simulink model "sm_car_4post_testrig"  (R2021b)
settings: Solver=ode23t  StartTime=0.0  StopTime=20  MaxStep=0.4  RelTol=1e-3  AbsTol=1e-3  EnableMultiTasking=on
PreLoadFcn:
  | sm_car_4post_param
  | sm_car_4post_param_posts
  | load sm_car_4post_op_01
  | load sm_car_4post_op_02
  | load sm_car_4post_op_03
  | 
  | 
  | sm_car_4post_vehicle_01_data
  | sm_car_4post_vehicle_02_data
  | sm_car_4post_vehicle_03_data
  | sm_car_4post_init_data
  | Vehicle = Vehicle_01;
  | sm_car_4post_op = sm_car_4post_op_01;
values from neighbouring files (symbols this model uses):
  brake_pressure_factor = 0.1    [sm_car_4post_param.m]
  brake_rear_factor = 0.3    [sm_car_4post_param.m]
  Init = struct    [sm_car_4post_init_data.m]
  N = 100    [sm_extr_data_cam_roller_curve.m]
  s = sin(q)    [sm_extr_data_cam_roller_curve.m]
  sm_car_4post_op_01 = simscape.op.create(simlog_sm_car_4post,20)    [sm_car_4post_gen_op.m]
  Vehicle_01 = struct    [sm_car_4post_vehicle_01_data.m]
undefined symbols (not defined in the file or in its folder): Axle, Hub, ShaftF, ShaftR, smcar_param, X, xy_data_car_side, xy_data_membrane, Y, Z
libraries: fl_lib x68, sm_lib x50, nesl_utility x40, sm_car_4post_lib x34, simulink x2
(part 3 of 4)

== system sm_car_4post_testrig/Vehicle/Chassis/Body ==
  Body Geometry : Subsystem  mask(Car Body Geometry){whl_cutout_rad=whl_cutout_rad, whl_base=whl_base, thk_top=thk_top, thk_side=thk_side, car_track=car_track, extr_data_emblem_f=extr_data_emblem_f, extr_data_emblem_r=extr_data_emblem_r, clr_body_geo_top=clr_body_geo_top, opc_body_geo_top=opc_body_geo_top, clr_body_geo_left=clr_body_geo_left, opc_body_geo_left=opc_body_geo_left, clr_body_geo_right=clr_body_geo_right, opc_body_geo_right=opc_body_geo_right, clr_emblem_f=clr_emblem_f, opc_emblem_f=opc_emblem_f, clr_emblem_r=clr_emblem_r, opc_emblem_r=opc_emblem_r}
      mask prompts: whl_cutout_rad "Wheel Cutout Radius (m)"; whl_base "Wheelbase (m)"; thk_top "Top Thickness (m)"; thk_side "Side Thickness (m)"; car_track "Width (m)"; extr_data_emblem_f "Emblem Data Front [xy] (m)"; extr_data_emblem_r "Emblem Data Rear [xy] (m)"
      mask help: Creates simple car geometry. Adjusting the wheel cutout radius and wheelbase causes the profile to be adjusted. Press the Plot Profile button to see how the parameters affect the profile.
      mask init:
      | [xy_data_car_top xy_data_car_side] = sm_extr_data_car_profile(whl_cutout_rad, whl_base,thk_top);
      mask TypeOptions extr_data_emblem_f:
      | Ornament
      | Front/ExtrusionCrossSection
      mask TypeOptions extr_data_emblem_r:
      | Ornament
      | Rear/ExtrusionCrossSection
      mask TypeOptions clr_body_geo_top: Top Surface/GraphicDiffuseColor
      mask TypeOptions opc_body_geo_top: Top Surface/GraphicOpacity
      mask TypeOptions clr_body_geo_left: Left Face/GraphicDiffuseColor
      mask TypeOptions opc_body_geo_left: Left Face/GraphicOpacity
      mask TypeOptions clr_body_geo_right: Right Face/GraphicDiffuseColor
      mask TypeOptions opc_body_geo_right: Right Face/GraphicOpacity
      mask TypeOptions clr_emblem_f:
      | Ornament
      | Front/GraphicDiffuseColor
      mask TypeOptions opc_emblem_f:
      | Ornament
      | Front/GraphicOpacity
      mask TypeOptions clr_emblem_r:
      | Ornament
      | Rear/GraphicDiffuseColor
      mask TypeOptions opc_emblem_r:
      | Ornament
      | Rear/GraphicOpacity
      mask DialogControl cont_geometry Prompt: Body Geometry
      mask DialogControl push_plot_profile Prompt: Plot Profile
      mask DialogControl push_plot_profile Callback:
      | v = get_param(gcb,'MaskWSVariables');
      | getMaskValue = containers.Map({v.Name}',{v.Value}');
      | evalin('base',...
      |     sprintf('sm_extr_data_car_profile(%s,%s,%s,''%s'');',...
      |     num2str(getMaskValue('whl_cutout_rad')),...
      |     num2str(getMaskValue('whl_base')),...
      |     num2str(getMaskValue('thk_top')),'plot'));
      mask DialogControl cont_emblem Prompt: Emblem
      mask DialogControl cont_vis Prompt: Visualization
      mask DialogControl text_vis_clr Prompt: Color [RGB]
      mask DialogControl text_vis_opc Prompt: Opac. (0-1)
      mask DialogControl text_vis_top Prompt: Top
      mask DialogControl text_vis_left Prompt: Left Side
      mask DialogControl text_vis_right Prompt: Right Side
      mask DialogControl text_vis_emblem_f Prompt: Emblem Front
      mask DialogControl text_vis_emblem_r Prompt: Emblem Rear
  Body Mass and Inertia : sm_lib/Body Elements/Spherical Solid  GraphicAmbientColor=[0.15 0.15 0.15 1.0]  BasedOnType=Density  CenterOfMass=[0 0 0]  CenterOfMassUnits=m  GraphicDiffuseColor=clr_chassis_hp_cg  Density=312*0.6  DensityUnits=kg/m^3  DoExposeReferenceFrame=on  GraphicEmissiveColor=[0.0 0.0 0.0 1.0]  ExportEntireGeometry=off  SerializedExposedGeometries=<ExposedGeometries/>  SerializedFrames=<Frames/>  MarkerShape=Sphere  MarkerSize=10  GraphicType=FromGeometry  InertiaType=Custom  Mass=chassis_mass  MassUnits=kg  MomentsOfInertia=chassis_inertia  MomentsOfInertiaUnits=kg*m^2  GraphicOpacity=opc_chassis_hp_cg  ProductsOfInertia=[0 0 0]  ProductsOfInertiaUnits=kg*m^2  GraphicShininess=75  GraphicSpecularColor=[0.5 0.5 0.5 1.0]  SphereRadius=size_chassis_hp_cg  SphereRadiusUnits=m  GraphicVisPropType=SimpleVisualProperties
  Transform Body : sm_lib/Frames and Transforms/Rigid Transform  TranslationMethod=Cartesian  TranslationStandardOffset=0.4225-0.1  TranslationLengthUnit=m  TranslationStandardAxis=+Z  TranslationCartesianOffset=body_geo_hp  TranslationROffset=0  TranslationROffsetUnits=m  TranslationZOffset=0  TranslationZOffsetUnits=m  TranslationThetaOffset=0  TranslationThetaOffsetUnits=deg  RotationMethod=None  RotationAngleUnits=deg  RotationStandardAxis=+Z  RotationAngle=0.0  RotationArbitraryAxis=[0 0 1]  FollAlignAxisA=+X  BaseAlignAxisA=+Y  FollAlignAxisB=+Y  BaseAlignAxisB=+Z  RotationSequenceAxes=FollowerAxes  RotationSequence=XYX  RotationSequenceAngles=[0 0 0]  RotationSequenceAnglesUnits=deg  RotationMatrix=[1 0 0; 0 1 0; 0 0 1]
  Transform Body CG : sm_lib/Frames and Transforms/Rigid Transform  TranslationMethod=Cartesian  TranslationStandardOffset=0  TranslationLengthUnit=m  TranslationStandardAxis=+Z  TranslationCartesianOffset=hp_chassis_cg  TranslationROffset=0  TranslationROffsetUnits=m  TranslationZOffset=0  TranslationZOffsetUnits=m  TranslationThetaOffset=0  TranslationThetaOffsetUnits=deg  RotationMethod=None  RotationAngleUnits=deg  RotationStandardAxis=+Z  RotationAngle=0.0  RotationArbitraryAxis=[0 0 1]  FollAlignAxisA=+X  BaseAlignAxisA=+Y  FollAlignAxisB=+Y  BaseAlignAxisB=+Z  RotationSequenceAxes=FollowerAxes  RotationSequence=XYX  RotationSequenceAngles=[0 0 0]  RotationSequenceAnglesUnits=deg  RotationMatrix=[1 0 0; 0 1 0; 0 0 1]
  Transform Front Mount : sm_lib/Frames and Transforms/Rigid Transform  TranslationMethod=Cartesian  TranslationStandardOffset=0  TranslationLengthUnit=m  TranslationStandardAxis=+X  TranslationCartesianOffset=hp_mount_fa  TranslationROffset=0  TranslationROffsetUnits=m  TranslationZOffset=0  TranslationZOffsetUnits=m  TranslationThetaOffset=0  TranslationThetaOffsetUnits=deg  RotationMethod=None  RotationAngleUnits=deg  RotationStandardAxis=+Z  RotationAngle=0.0  RotationArbitraryAxis=[0 0 1]  FollAlignAxisA=+X  BaseAlignAxisA=+Y  FollAlignAxisB=+Y  BaseAlignAxisB=+Z  RotationSequenceAxes=FollowerAxes  RotationSequence=XYX  RotationSequenceAngles=[0 0 0]  RotationSequenceAnglesUnits=deg  RotationMatrix=[1 0 0; 0 1 0; 0 0 1]
  Transform Power Mount : sm_lib/Frames and Transforms/Rigid Transform  TranslationMethod=Cartesian  TranslationStandardOffset=0  TranslationLengthUnit=m  TranslationStandardAxis=+Z  TranslationCartesianOffset=hp_mount_power  TranslationROffset=0  TranslationROffsetUnits=m  TranslationZOffset=0  TranslationZOffsetUnits=m  TranslationThetaOffset=0  TranslationThetaOffsetUnits=deg  RotationMethod=None  RotationAngleUnits=deg  RotationStandardAxis=+Z  RotationAngle=0.0  RotationArbitraryAxis=[0 0 1]  FollAlignAxisA=+X  BaseAlignAxisA=+Y  FollAlignAxisB=+Y  BaseAlignAxisB=+Z  RotationSequenceAxes=FollowerAxes  RotationSequence=XYX  RotationSequenceAngles=[0 0 0]  RotationSequenceAnglesUnits=deg  RotationMatrix=[1 0 0; 0 1 0; 0 0 1]
  Transform Rear Mount : sm_lib/Frames and Transforms/Rigid Transform  TranslationMethod=Cartesian  TranslationStandardOffset=0  TranslationLengthUnit=m  TranslationStandardAxis=-X  TranslationCartesianOffset=hp_mount_ra  TranslationROffset=0  TranslationROffsetUnits=m  TranslationZOffset=0  TranslationZOffsetUnits=m  TranslationThetaOffset=0  TranslationThetaOffsetUnits=deg  RotationMethod=None  RotationAngleUnits=deg  RotationStandardAxis=+Z  RotationAngle=0.0  RotationArbitraryAxis=[0 0 1]  FollAlignAxisA=+X  BaseAlignAxisA=+Y  FollAlignAxisB=+Y  BaseAlignAxisB=+Z  RotationSequenceAxes=FollowerAxes  RotationSequence=XYX  RotationSequenceAngles=[0 0 0]  RotationSequenceAnglesUnits=deg  RotationMatrix=[1 0 0; 0 1 0; 0 0 1]
  Vis HP Mount Front : sm_lib/Body Elements/Spherical Solid  GraphicAmbientColor=[0.15 0.15 0.15 1.0]  BasedOnType=Density  CenterOfMass=[0 0 0]  CenterOfMassUnits=m  GraphicDiffuseColor=clr_chassis_hp_cg  Density=312*0.6  DensityUnits=kg/m^3  DoExposeReferenceFrame=on  GraphicEmissiveColor=[0.0 0.0 0.0 1.0]  ExportEntireGeometry=off  SerializedExposedGeometries=<ExposedGeometries/>  SerializedFrames=<Frames/>  MarkerShape=Sphere  MarkerSize=10  GraphicType=FromGeometry  InertiaType=PointMass  Mass=0  MassUnits=kg  MomentsOfInertia=[1 1 1]  MomentsOfInertiaUnits=kg*m^2  GraphicOpacity=opc_chassis_hp_cg  ProductsOfInertia=[0 0 0]  ProductsOfInertiaUnits=kg*m^2  GraphicShininess=75  GraphicSpecularColor=[0.5 0.5 0.5 1.0]  SphereRadius=size_chassis_hp_cg  SphereRadiusUnits=m  GraphicVisPropType=SimpleVisualProperties
  Vis HP Mount Rear : sm_lib/Body Elements/Spherical Solid  GraphicAmbientColor=[0.15 0.15 0.15 1.0]  BasedOnType=Density  CenterOfMass=[0 0 0]  CenterOfMassUnits=m  GraphicDiffuseColor=clr_chassis_hp_cg  Density=312*0.6  DensityUnits=kg/m^3  DoExposeReferenceFrame=on  GraphicEmissiveColor=[0.0 0.0 0.0 1.0]  ExportEntireGeometry=off  SerializedExposedGeometries=<ExposedGeometries/>  SerializedFrames=<Frames/>  MarkerShape=Sphere  MarkerSize=10  GraphicType=FromGeometry  InertiaType=PointMass  Mass=0  MassUnits=kg  MomentsOfInertia=[1 1 1]  MomentsOfInertiaUnits=kg*m^2  GraphicOpacity=opc_chassis_hp_cg  ProductsOfInertia=[0 0 0]  ProductsOfInertiaUnits=kg*m^2  GraphicShininess=75  GraphicSpecularColor=[0.5 0.5 0.5 1.0]  SphereRadius=size_chassis_hp_cg  SphereRadiusUnits=m  GraphicVisPropType=SimpleVisualProperties
  FA : PMIOPort  Side=Right
  Power : PMIOPort  Port=2  Side=Right
  W : PMIOPort  Port=3  Side=Left
  RA : PMIOPort  Port=4  Side=Right
  connections:
  Power/RConn1 -- Transform Power Mount/RConn1
  Transform Rear Mount/RConn1 -- Vis HP Mount Rear/RConn1 -- RA/RConn1
  FA/RConn1 -- Transform Front Mount/RConn1 -- Vis HP Mount Front/RConn1
  Body Mass and Inertia/RConn1 -- Transform Body CG/RConn1
  Transform Rear Mount/LConn1 -- Transform Power Mount/LConn1 -- Transform Front Mount/LConn1 -- W/RConn1 -- Transform Body CG/LConn1 -- Transform Body/LConn1
  Body Geometry/LConn1 -- Transform Body/RConn1

== system sm_car_4post_testrig/Vehicle/Chassis/Dampers ==
  Ctrl : Inport
  Independent : Subsystem  VariantControl=Independent
  FL : PMIOPort  Side=Left
  FR : PMIOPort  Port=2  Side=Right
  RL : PMIOPort  Port=3  Side=Left
  RR : PMIOPort  Port=4  Side=Right
  meas : Outport  VectorParamsAs1DForOutWhenUnconnected=off
  wires:
  Independent/1(meas) -> meas/1
  Ctrl/1 -> Independent/1(Ctrl)
  connections:
  Independent/RConn2 -- RR/RConn1
  Independent/RConn1 -- FR/RConn1
  Independent/LConn2 -- RL/RConn1
  Independent/LConn1 -- FL/RConn1

== system sm_car_4post_testrig/Vehicle/Chassis/Springs ==
  Ctrl : Inport
  Independent : Subsystem  VariantControl=Independent
  FL : PMIOPort  Side=Left
  FR : PMIOPort  Port=2  Side=Right
  RL : PMIOPort  Port=3  Side=Left
  RR : PMIOPort  Port=4  Side=Right
  meas : Outport  VectorParamsAs1DForOutWhenUnconnected=off
  wires:
  Independent/1(meas) -> meas/1
  Ctrl/1 -> Independent/1(Ctrl)
  connections:
  Independent/RConn2 -- RR/RConn1
  Independent/RConn1 -- FR/RConn1
  Independent/LConn1 -- FL/RConn1
  Independent/LConn2 -- RL/RConn1

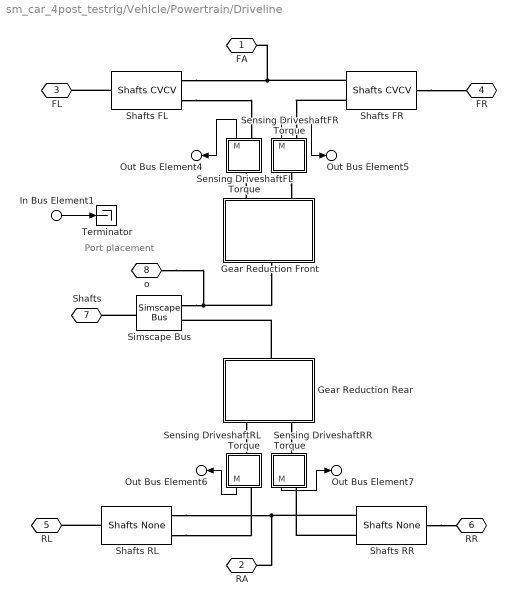
== system sm_car_4post_testrig/Vehicle/Powertrain/Driveline ==
  note: Port placement
  In Bus Element1 : Inport  PortName=CtrlBus
  Gear Reduction Front : Subsystem
  Gear Reduction Rear : Subsystem
  Sensing DriveshaftFL Torque : Subsystem
  Sensing DriveshaftFR Torque : Subsystem
  Sensing DriveshaftRL Torque : Subsystem
  Sensing DriveshaftRR Torque : Subsystem
  Shafts FL : sm_car_4post_lib/Shafts CVCV  popup_leftRight=Left  Shaft=Driveline.ShaftsFL
      settings: SourceProductBaseCode=MS
  Shafts FR : sm_car_4post_lib/Shafts CVCV  popup_leftRight=Right  Shaft=Driveline.ShaftsFR
      settings: SourceProductBaseCode=MS
  Shafts RL : sm_car_4post_lib/Shafts None  popup_leftRight=Left  Shaft=Driveline.ShaftsRL
      settings: SourceProductBaseCode=MS
  Shafts RR : sm_car_4post_lib/Shafts None  popup_leftRight=Right  Shaft=Driveline.ShaftsRR
      settings: SourceProductBaseCode=MS
  Simscape Bus : SimscapeBus  HierarchyStrings=ShaftF;ShaftR
  Terminator : Terminator
  FA : PMIOPort  Side=Left
  RA : PMIOPort  Port=2  Side=Right
  FL : PMIOPort  Port=3  Side=Left
  FR : PMIOPort  Port=4  Side=Right
  RL : PMIOPort  Port=5  Side=Left
  RR : PMIOPort  Port=6  Side=Right
  Shafts : PMIOPort  Port=7  Side=Left
  o : PMIOPort  Port=8  Side=Right
  Out Bus Element4 : Outport  VectorParamsAs1DForOutWhenUnconnected=off  PortName=DriveOut  Element=MDriveshaftFL
  Out Bus Element5 : Outport  VectorParamsAs1DForOutWhenUnconnected=off  PortName=DriveOut  Element=MDriveshaftFR
  Out Bus Element6 : Outport  VectorParamsAs1DForOutWhenUnconnected=off  PortName=DriveOut  Element=MDriveshaftRL
  Out Bus Element7 : Outport  VectorParamsAs1DForOutWhenUnconnected=off  PortName=DriveOut  Element=MDriveshaftRR
  wires:
  Sensing DriveshaftFR Torque/1(M) -> Out Bus Element5/1
  Sensing DriveshaftFL Torque/1(M) -> Out Bus Element4/1
  Sensing DriveshaftRL Torque/1(M) -> Out Bus Element6/1
  Sensing DriveshaftRR Torque/1(M) -> Out Bus Element7/1
  In Bus Element1/1 -> Terminator/1
  connections:
  Shafts FL/RConn1 -- Shafts FR/RConn1 -- FA/RConn1
  Shafts FR/LConn1 -- FR/RConn1
  Shafts RR/LConn1 -- RR/RConn1
  Shafts RL/LConn1 -- RL/RConn1
  Shafts FL/LConn1 -- FL/RConn1
  Shafts FL/RConn2 -- Sensing DriveshaftFL Torque/RConn1
  Shafts RR/RConn2 -- Sensing DriveshaftRR Torque/RConn1
  Shafts RL/RConn2 -- Sensing DriveshaftRL Torque/RConn1
  Gear Reduction Rear/LConn1 -- Simscape Bus/LConn2
  Gear Reduction Rear/RConn2 -- Sensing DriveshaftRR Torque/LConn1
  Gear Reduction Rear/RConn1 -- Sensing DriveshaftRL Torque/LConn1
  Simscape Bus/RConn1 -- Shafts/RConn1
  Shafts RL/RConn1 -- Shafts RR/RConn1 -- RA/RConn1
  Shafts FR/RConn2 -- Sensing DriveshaftFR Torque/RConn1
  o/RConn1 -- Gear Reduction Front/LConn1 -- Simscape Bus/LConn1
  Gear Reduction Front/RConn1 -- Sensing DriveshaftFL Torque/LConn1
  Sensing DriveshaftFR Torque/LConn1 -- Gear Reduction Front/RConn2

== system sm_car_4post_testrig/Vehicle/Powertrain/Power ==
  CtrlBus : Inport
  IdealTwoMotor : Subsystem  VariantControl=IdealTwoMotor  mask(Two Motor){motor_ts_f=100, motor_ts_r=100}
      mask prompts: motor_ts_f "Front Motor Cutoff Frequency (Hz)"; motor_ts_r "Rear Motor Cutoff Frequency (Hz)"
      mask help: Models two independent motors as a torque source with a simple first-order lag.
  Shafts : PMIOPort  Side=Left
  Ref : PMIOPort  Port=2  Side=Right
  PowerOut : Outport  VectorParamsAs1DForOutWhenUnconnected=off
  wires:
  IdealTwoMotor/1(PowerOut) -> PowerOut/1
  CtrlBus/1 -> IdealTwoMotor/1(CtrlBus)
  connections:
  IdealTwoMotor/RConn1 -- Ref/RConn1
  IdealTwoMotor/LConn1 -- Shafts/RConn1

== system sm_car_4post_testrig/Vehicle/Body Sensor/Roll Pitch/Calculate aPitch ==
  Roll Angle : Inport
  uvec : Inport  Port=2
  Asin : Trigonometry  Operator=asin
  Cos : Trigonometry  Operator=cos
  Divide : Product  Inputs=*/
  Divide1 : Product  Inputs=*/
  Selector : Selector  InputPortWidth=3  IndexOptions=Index vector (dialog)  Indices=[3]  OutputSizes=1
  magnitude : Fcn  Expr=sqrt(u(1)*u(1)+u(2)*u(2)+u(3)*u(3))
  Angle : Outport  VectorParamsAs1DForOutWhenUnconnected=off
  wires:
  Divide1/1 -> Asin/1
  uvec/1 -> magnitude/1, Selector/1
  magnitude/1 -> Divide1/2
  Selector/1 -> Divide/1
  Roll Angle/1 -> Cos/1
  Asin/1 -> Angle/1
  Divide/1 -> Divide1/1
  Cos/1 -> Divide/2

== system sm_car_4post_testrig/Vehicle/Body Sensor/Roll Pitch/Calculate aRoll ==
  uvec : Inport
  Demux : Demux  Outputs=3
  Mux : Mux  Inputs=2
  Trigonometric Function1 : Trigonometry  Operator=atan2
  magnitude : Fcn  Expr=sqrt(u(1)*u(1)+u(2)*u(2))
  Angle : Outport  VectorParamsAs1DForOutWhenUnconnected=off
  wires:
  Demux/2 -> Mux/2
  magnitude/1 -> Trigonometric Function1/2
  Mux/1 -> magnitude/1
  Demux/3 -> Trigonometric Function1/1
  Trigonometric Function1/1 -> Angle/1
  uvec/1 -> Demux/1
  Demux/1 -> Mux/1

== system sm_car_4post_testrig/Vehicle/Brakes/Pedal/Actuator FL ==
  Apply : Inport
  Filter : TransferFcn  Numerator=brk_max_p  Denominator=[brk_filt 1]
  Simulink-PS Converter : nesl_utility/Simulink-PS Converter  PhysicalDomain=network_engine_domain  SubClassName=ps_input  LeftPortType=input  RightPortType=output  PseudoPeriodic=off  Frequencies=[]  NoiseDistribution=none  NoiseParameters=[]  Unit=1  AffineConversion=off  FilteringAndDerivatives=provide  SimscapeFilterOrder=1  InputFilterTimeConstant=0.001  UdotUserProvided=0
      settings: SourceProductBaseCode=PW,SS
  P : PMIOPort  Side=Right
  wires:
  Filter/1 -> Simulink-PS Converter/1
  Apply/1 -> Filter/1
  connections:
  Simulink-PS Converter/RConn1 -- P/RConn1

== system sm_car_4post_testrig/Vehicle/Brakes/Pedal/Actuator FR ==
  Apply : Inport
  Filter : TransferFcn  Numerator=brk_max_p  Denominator=[brk_filt 1]
  Simulink-PS Converter : nesl_utility/Simulink-PS Converter  PhysicalDomain=network_engine_domain  SubClassName=ps_input  LeftPortType=input  RightPortType=output  PseudoPeriodic=off  Frequencies=[]  NoiseDistribution=none  NoiseParameters=[]  Unit=1  AffineConversion=off  FilteringAndDerivatives=provide  SimscapeFilterOrder=1  InputFilterTimeConstant=0.001  UdotUserProvided=0
      settings: SourceProductBaseCode=PW,SS
  P : PMIOPort  Side=Right
  wires:
  Apply/1 -> Filter/1
  Filter/1 -> Simulink-PS Converter/1
  connections:
  Simulink-PS Converter/RConn1 -- P/RConn1

== system sm_car_4post_testrig/Vehicle/Brakes/Pedal/Actuator RL ==
  Apply : Inport
  Filter : TransferFcn  Numerator=brk_max_p  Denominator=[brk_filt 1]
  Simulink-PS Converter : nesl_utility/Simulink-PS Converter  PhysicalDomain=network_engine_domain  SubClassName=ps_input  LeftPortType=input  RightPortType=output  PseudoPeriodic=off  Frequencies=[]  NoiseDistribution=none  NoiseParameters=[]  Unit=1  AffineConversion=off  FilteringAndDerivatives=provide  SimscapeFilterOrder=1  InputFilterTimeConstant=0.001  UdotUserProvided=0
      settings: SourceProductBaseCode=PW,SS
  P : PMIOPort  Side=Right
  wires:
  Apply/1 -> Filter/1
  Filter/1 -> Simulink-PS Converter/1
  connections:
  Simulink-PS Converter/RConn1 -- P/RConn1

== system sm_car_4post_testrig/Vehicle/Brakes/Pedal/Actuator RR ==
  Apply : Inport
  Filter : TransferFcn  Numerator=brk_max_p  Denominator=[brk_filt 1]
  Simulink-PS Converter : nesl_utility/Simulink-PS Converter  PhysicalDomain=network_engine_domain  SubClassName=ps_input  LeftPortType=input  RightPortType=output  PseudoPeriodic=off  Frequencies=[]  NoiseDistribution=none  NoiseParameters=[]  Unit=1  AffineConversion=off  FilteringAndDerivatives=provide  SimscapeFilterOrder=1  InputFilterTimeConstant=0.001  UdotUserProvided=0
      settings: SourceProductBaseCode=PW,SS
  P : PMIOPort  Side=Right
  wires:
  Filter/1 -> Simulink-PS Converter/1
  Apply/1 -> Filter/1
  connections:
  Simulink-PS Converter/RConn1 -- P/RConn1

== system sm_car_4post_testrig/Vehicle/Brakes/Pedal/Brake FL ==
  note: Very basic implementation of a brake.
      | A more realistic brake is available in Simscape Driveline
  Ideal Rotational Motion Sensor : fl_lib/Mechanical/Mechanical Sensors/Ideal Rotational Motion Sensor  wrap_angle=simscape.enum.onoff.off  offset=0 rad
  Ideal Torque Source : fl_lib/Mechanical/Mechanical Sources/Ideal Torque Source
  Mechanical Rotational Reference : fl_lib/Mechanical/Rotational Elements/Mechanical Rotational Reference
  PS Gain : fl_lib/Physical Signals/Functions/PS Gain  gain=1 1/(rad/s)
  PS Gain1 : fl_lib/Physical Signals/Functions/PS Gain  gain=-1 N*m
  PS Gain2 : fl_lib/Physical Signals/Functions/PS Gain  gain=brake_pressure_factor
  PS Product : fl_lib/Physical Signals/Functions/PS Product
  PS Terminator : fl_lib/Physical Signals/Sinks/PS Terminator
  R : PMIOPort  Side=Left
  P : PMIOPort  Port=2  Side=Left
  connections:
  Ideal Rotational Motion Sensor/RConn3 -- PS Terminator/LConn1
  PS Gain2/LConn1 -- P/RConn1
  Ideal Rotational Motion Sensor/RConn2 -- PS Gain/LConn1
  PS Gain1/LConn1 -- PS Product/RConn1
  R/RConn1 -- Ideal Rotational Motion Sensor/LConn1 -- Ideal Torque Source/LConn1
  Ideal Rotational Motion Sensor/RConn1 -- Mechanical Rotational Reference/LConn1 -- Ideal Torque Source/RConn2
  PS Gain/RConn1 -- PS Product/LConn2
  Ideal Torque Source/RConn1 -- PS Gain1/RConn1
  PS Product/LConn1 -- PS Gain2/RConn1

== system sm_car_4post_testrig/Vehicle/Brakes/Pedal/Brake FR ==
  note: Very basic implementation of a brake.
      | A more realistic brake is available in Simscape Driveline
  Ideal Rotational Motion Sensor : fl_lib/Mechanical/Mechanical Sensors/Ideal Rotational Motion Sensor  wrap_angle=simscape.enum.onoff.off  offset=0 rad
  Ideal Torque Source : fl_lib/Mechanical/Mechanical Sources/Ideal Torque Source
  Mechanical Rotational Reference : fl_lib/Mechanical/Rotational Elements/Mechanical Rotational Reference
  PS Gain : fl_lib/Physical Signals/Functions/PS Gain  gain=1 1/(rad/s)
  PS Gain1 : fl_lib/Physical Signals/Functions/PS Gain  gain=-1 N*m
  PS Gain2 : fl_lib/Physical Signals/Functions/PS Gain  gain=brake_pressure_factor
  PS Product : fl_lib/Physical Signals/Functions/PS Product
  PS Terminator : fl_lib/Physical Signals/Sinks/PS Terminator
  P : PMIOPort  Side=Left
  R : PMIOPort  Port=2  Side=Left
  connections:
  Ideal Torque Source/RConn1 -- PS Gain1/RConn1
  PS Gain/RConn1 -- PS Product/LConn2
  Mechanical Rotational Reference/LConn1 -- Ideal Torque Source/RConn2 -- Ideal Rotational Motion Sensor/RConn1
  Ideal Torque Source/LConn1 -- Ideal Rotational Motion Sensor/LConn1 -- R/RConn1
  PS Gain1/LConn1 -- PS Product/RConn1
  Ideal Rotational Motion Sensor/RConn2 -- PS Gain/LConn1
  PS Gain2/LConn1 -- P/RConn1
  Ideal Rotational Motion Sensor/RConn3 -- PS Terminator/LConn1
  PS Product/LConn1 -- PS Gain2/RConn1

== system sm_car_4post_testrig/Vehicle/Brakes/Pedal/Brake RL ==
  note: Very basic implementation of a brake.
      | A more realistic brake is available in Simscape Driveline
  Ideal Rotational Motion Sensor : fl_lib/Mechanical/Mechanical Sensors/Ideal Rotational Motion Sensor  wrap_angle=simscape.enum.onoff.off  offset=0 rad
  Ideal Torque Source : fl_lib/Mechanical/Mechanical Sources/Ideal Torque Source
  Mechanical Rotational Reference : fl_lib/Mechanical/Rotational Elements/Mechanical Rotational Reference
  PS Gain : fl_lib/Physical Signals/Functions/PS Gain  gain=1 1/(rad/s)
  PS Gain1 : fl_lib/Physical Signals/Functions/PS Gain  gain=-1 N*m
  PS Gain2 : fl_lib/Physical Signals/Functions/PS Gain  gain=brake_pressure_factor*brake_rear_factor
  PS Product : fl_lib/Physical Signals/Functions/PS Product
  PS Terminator : fl_lib/Physical Signals/Sinks/PS Terminator
  R : PMIOPort  Side=Left
  P : PMIOPort  Port=2  Side=Left
  connections:
  Ideal Torque Source/RConn1 -- PS Gain1/RConn1
  PS Gain/RConn1 -- PS Product/LConn2
  Ideal Torque Source/RConn2 -- Mechanical Rotational Reference/LConn1 -- Ideal Rotational Motion Sensor/RConn1
  Ideal Torque Source/LConn1 -- Ideal Rotational Motion Sensor/LConn1 -- R/RConn1
  PS Gain1/LConn1 -- PS Product/RConn1
  Ideal Rotational Motion Sensor/RConn2 -- PS Gain/LConn1
  PS Product/LConn1 -- PS Gain2/RConn1
  Ideal Rotational Motion Sensor/RConn3 -- PS Terminator/LConn1
  PS Gain2/LConn1 -- P/RConn1

== system sm_car_4post_testrig/Vehicle/Brakes/Pedal/Brake RR ==
  note: Very basic implementation of a brake.
      | A more realistic brake is available in Simscape Driveline
  Ideal Rotational Motion Sensor : fl_lib/Mechanical/Mechanical Sensors/Ideal Rotational Motion Sensor  wrap_angle=simscape.enum.onoff.off  offset=0 rad
  Ideal Torque Source : fl_lib/Mechanical/Mechanical Sources/Ideal Torque Source
  Mechanical Rotational Reference : fl_lib/Mechanical/Rotational Elements/Mechanical Rotational Reference
  PS Gain : fl_lib/Physical Signals/Functions/PS Gain  gain=1 1/(rad/s)
  PS Gain1 : fl_lib/Physical Signals/Functions/PS Gain  gain=-1 N*m
  PS Gain2 : fl_lib/Physical Signals/Functions/PS Gain  gain=brake_pressure_factor*brake_rear_factor
  PS Product : fl_lib/Physical Signals/Functions/PS Product
  PS Terminator : fl_lib/Physical Signals/Sinks/PS Terminator
  P : PMIOPort  Side=Left
  R : PMIOPort  Port=2  Side=Left
  connections:
  Ideal Rotational Motion Sensor/RConn3 -- PS Terminator/LConn1
  PS Gain2/LConn1 -- P/RConn1
  Ideal Rotational Motion Sensor/RConn2 -- PS Gain/LConn1
  PS Gain1/LConn1 -- PS Product/RConn1
  R/RConn1 -- Ideal Rotational Motion Sensor/LConn1 -- Ideal Torque Source/LConn1
  Ideal Rotational Motion Sensor/RConn1 -- Ideal Torque Source/RConn2 -- Mechanical Rotational Reference/LConn1
  PS Gain/RConn1 -- PS Product/LConn2
  Ideal Torque Source/RConn1 -- PS Gain1/RConn1
  PS Product/LConn1 -- PS Gain2/RConn1

== system sm_car_4post_testrig/Vehicle/Brakes/Pedal/Sensing Torque FL ==
  Ideal Torque Sensor : fl_lib/Mechanical/Mechanical Sensors/Ideal Torque Sensor
  PS-Simulink Converter : nesl_utility/PS-Simulink Converter  PhysicalDomain=network_engine_domain  SubClassName=ps_output  LeftPortType=input  RightPortType=output  PseudoPeriodic=off  Frequencies=[]  Unit=N*m  AffineConversion=off
      settings: SourceProductBaseCode=PW,SS
  C : PMIOPort  Side=Right
  R : PMIOPort  Port=2  Side=Left
  T : Outport  VectorParamsAs1DForOutWhenUnconnected=off
  wires:
  PS-Simulink Converter/1 -> T/1
  connections:
  PS-Simulink Converter/LConn1 -- Ideal Torque Sensor/RConn2
  Ideal Torque Sensor/RConn1 -- C/RConn1
  Ideal Torque Sensor/LConn1 -- R/RConn1

== system sm_car_4post_testrig/Vehicle/Brakes/Pedal/Sensing Torque FR ==
  Ideal Torque Sensor : fl_lib/Mechanical/Mechanical Sensors/Ideal Torque Sensor
  PS-Simulink Converter : nesl_utility/PS-Simulink Converter  PhysicalDomain=network_engine_domain  SubClassName=ps_output  LeftPortType=input  RightPortType=output  PseudoPeriodic=off  Frequencies=[]  Unit=N*m  AffineConversion=off
      settings: SourceProductBaseCode=PW,SS
  C : PMIOPort  Side=Right
  R : PMIOPort  Port=2  Side=Left
  T : Outport  VectorParamsAs1DForOutWhenUnconnected=off
  wires:
  PS-Simulink Converter/1 -> T/1
  connections:
  Ideal Torque Sensor/LConn1 -- R/RConn1
  Ideal Torque Sensor/RConn1 -- C/RConn1
  PS-Simulink Converter/LConn1 -- Ideal Torque Sensor/RConn2

== system sm_car_4post_testrig/Vehicle/Brakes/Pedal/Sensing Torque RL ==
  Ideal Torque Sensor : fl_lib/Mechanical/Mechanical Sensors/Ideal Torque Sensor
  PS-Simulink Converter : nesl_utility/PS-Simulink Converter  PhysicalDomain=network_engine_domain  SubClassName=ps_output  LeftPortType=input  RightPortType=output  PseudoPeriodic=off  Frequencies=[]  Unit=N*m  AffineConversion=off
      settings: SourceProductBaseCode=PW,SS
  C : PMIOPort  Side=Right
  R : PMIOPort  Port=2  Side=Left
  T : Outport  VectorParamsAs1DForOutWhenUnconnected=off
  wires:
  PS-Simulink Converter/1 -> T/1
  connections:
  PS-Simulink Converter/LConn1 -- Ideal Torque Sensor/RConn2
  Ideal Torque Sensor/RConn1 -- C/RConn1
  Ideal Torque Sensor/LConn1 -- R/RConn1

== system sm_car_4post_testrig/Vehicle/Brakes/Pedal/Sensing Torque RR ==
  Ideal Torque Sensor : fl_lib/Mechanical/Mechanical Sensors/Ideal Torque Sensor
  PS-Simulink Converter : nesl_utility/PS-Simulink Converter  PhysicalDomain=network_engine_domain  SubClassName=ps_output  LeftPortType=input  RightPortType=output  PseudoPeriodic=off  Frequencies=[]  Unit=N*m  AffineConversion=off
      settings: SourceProductBaseCode=PW,SS
  C : PMIOPort  Side=Right
  R : PMIOPort  Port=2  Side=Left
  T : Outport  VectorParamsAs1DForOutWhenUnconnected=off
  wires:
  PS-Simulink Converter/1 -> T/1
  connections:
  Ideal Torque Sensor/LConn1 -- R/RConn1
  Ideal Torque Sensor/RConn1 -- C/RConn1
  PS-Simulink Converter/LConn1 -- Ideal Torque Sensor/RConn2

== system sm_car_4post_testrig/Vehicle/Chassis/Body/Body Geometry ==
  Left Face : sm_lib/Body Elements/Extruded Solid  GraphicAmbientColor=[0.15 0.15 0.15 1.0]  BasedOnType=Density  CenterOfMass=[0 0 0]  CenterOfMassUnits=m  GraphicDiffuseColor=clr_body_geo_left  ExportConvexHullGeometry=off  ExtrusionCrossSection=xy_data_car_side  ExtrusionCrossSectionUnits=m  Density=1000  DensityUnits=kg/m^3  DoExposeReferenceFrame=on  GraphicEmissiveColor=[0.0 0.0 0.0 1.0]  ExportEntireGeometry=off  ExtrusionLength=thk_side  ExtrusionLengthUnits=m  ExtrusionType=General  SerializedFrames=<Frames/>  MarkerShape=Sphere  MarkerSize=10  GraphicType=FromGeometry  InertiaType=PointMass  Mass=0  MassUnits=kg  MomentsOfInertia=[1 1 1]  MomentsOfInertiaUnits=kg*m^2  PolygonNumSides=3  GraphicOpacity=opc_body_geo_left  PolygonOuterRadius=1  PolygonOuterRadiusUnits=m  ProductsOfInertia=[0 0 0]  ProductsOfInertiaUnits=kg*m^2  GraphicShininess=75  GraphicSpecularColor=[0.5 0.5 0.5 1.0]  GraphicVisPropType=SimpleVisualProperties
  Ornament Front : sm_lib/Body Elements/Extruded Solid  GraphicAmbientColor=[0.15 0.15 0.15 1.0]  BasedOnType=Density  CenterOfMass=[0 0 0]  CenterOfMassUnits=m  GraphicDiffuseColor=clr_emblem_f  ExportConvexHullGeometry=off  ExtrusionCrossSection=extr_data_emblem_f  ExtrusionCrossSectionUnits=m  Density=1000  DensityUnits=kg/m^3  DoExposeReferenceFrame=on  GraphicEmissiveColor=[0.0 0.0 0.0 1.0]  ExportEntireGeometry=off  ExtrusionLength=0.01  ExtrusionLengthUnits=m  ExtrusionType=General  SerializedFrames=<Frames/>  MarkerShape=Sphere  MarkerSize=10  GraphicType=FromGeometry  InertiaType=CalculateFromGeometry  Mass=1  MassUnits=kg  MomentsOfInertia=[1 1 1]  MomentsOfInertiaUnits=kg*m^2  PolygonNumSides=3  GraphicOpacity=opc_emblem_f  PolygonOuterRadius=1  PolygonOuterRadiusUnits=m  ProductsOfInertia=[0 0 0]  ProductsOfInertiaUnits=kg*m^2  GraphicShininess=75  GraphicSpecularColor=[0.5 0.5 0.5 1.0]  GraphicVisPropType=SimpleVisualProperties
  Ornament Rear : sm_lib/Body Elements/Extruded Solid  GraphicAmbientColor=[0.15 0.15 0.15 1.0]  BasedOnType=Density  CenterOfMass=[0 0 0]  CenterOfMassUnits=m  GraphicDiffuseColor=clr_emblem_r  ExportConvexHullGeometry=off  ExtrusionCrossSection=extr_data_emblem_r  ExtrusionCrossSectionUnits=m  Density=1000  DensityUnits=kg/m^3  DoExposeReferenceFrame=on  GraphicEmissiveColor=[0.0 0.0 0.0 1.0]  ExportEntireGeometry=off  ExtrusionLength=0.01  ExtrusionLengthUnits=m  ExtrusionType=General  SerializedFrames=<Frames/>  MarkerShape=Sphere  MarkerSize=10  GraphicType=FromGeometry  InertiaType=CalculateFromGeometry  Mass=1  MassUnits=kg  MomentsOfInertia=[1 1 1]  MomentsOfInertiaUnits=kg*m^2  PolygonNumSides=3  GraphicOpacity=opc_emblem_r  PolygonOuterRadius=1  PolygonOuterRadiusUnits=m  ProductsOfInertia=[0 0 0]  ProductsOfInertiaUnits=kg*m^2  GraphicShininess=75  GraphicSpecularColor=[0.5 0.5 0.5 1.0]  GraphicVisPropType=SimpleVisualProperties
  Right Face : sm_lib/Body Elements/Extruded Solid  GraphicAmbientColor=[0.15 0.15 0.15 1.0]  BasedOnType=Density  CenterOfMass=[0 0 0]  CenterOfMassUnits=m  GraphicDiffuseColor=clr_body_geo_right  ExportConvexHullGeometry=off  ExtrusionCrossSection=xy_data_car_side  ExtrusionCrossSectionUnits=m  Density=1000  DensityUnits=kg/m^3  DoExposeReferenceFrame=on  GraphicEmissiveColor=[0.0 0.0 0.0 1.0]  ExportEntireGeometry=off  ExtrusionLength=thk_side  ExtrusionLengthUnits=m  ExtrusionType=General  SerializedFrames=<Frames/>  MarkerShape=Sphere  MarkerSize=10  GraphicType=FromGeometry  InertiaType=PointMass  Mass=0  MassUnits=kg  MomentsOfInertia=[1 1 1]  MomentsOfInertiaUnits=kg*m^2  PolygonNumSides=3  GraphicOpacity=opc_body_geo_right  PolygonOuterRadius=1  PolygonOuterRadiusUnits=m  ProductsOfInertia=[0 0 0]  ProductsOfInertiaUnits=kg*m^2  GraphicShininess=75  GraphicSpecularColor=[0.5 0.5 0.5 1.0]  GraphicVisPropType=SimpleVisualProperties
  Top Surface : sm_lib/Body Elements/Extruded Solid  GraphicAmbientColor=[0.15 0.15 0.15 1.0]  BasedOnType=Density  CenterOfMass=[0 0 0]  CenterOfMassUnits=m  GraphicDiffuseColor=clr_body_geo_top  ExportConvexHullGeometry=off  ExtrusionCrossSection=xy_data_car_top  ExtrusionCrossSectionUnits=m  Density=0  DensityUnits=kg/m^3  DoExposeReferenceFrame=on  GraphicEmissiveColor=[0.0 0.0 0.0 1.0]  ExportEntireGeometry=off  ExtrusionLength=car_track  ExtrusionLengthUnits=m  ExtrusionType=General  SerializedFrames=<Frames/>  MarkerShape=Sphere  MarkerSize=10  GraphicType=FromGeometry  InertiaType=PointMass  Mass=0  MassUnits=kg  MomentsOfInertia=[1 1 1]  MomentsOfInertiaUnits=kg*m^2  PolygonNumSides=3  GraphicOpacity=opc_body_geo_top  PolygonOuterRadius=1  PolygonOuterRadiusUnits=m  ProductsOfInertia=[0 0 0]  ProductsOfInertiaUnits=kg*m^2  GraphicShininess=75  GraphicSpecularColor=[0.5 0.5 0.5 1.0]  GraphicVisPropType=SimpleVisualProperties
  Transform Extrusion Axes : sm_lib/Frames and Transforms/Rigid Transform  TranslationMethod=None  TranslationStandardOffset=0  TranslationLengthUnit=m  TranslationStandardAxis=+Z  TranslationCartesianOffset=[0 0 0]  TranslationROffset=0  TranslationROffsetUnits=m  TranslationZOffset=0  TranslationZOffsetUnits=m  TranslationThetaOffset=0  TranslationThetaOffsetUnits=deg  RotationMethod=StandardAxis  RotationAngleUnits=deg  RotationStandardAxis=+X  RotationAngle=90  RotationArbitraryAxis=[0 0 1]  FollAlignAxisA=+X  BaseAlignAxisA=+Y  FollAlignAxisB=+Y  BaseAlignAxisB=+Z  RotationSequenceAxes=FollowerAxes  RotationSequence=XYX  RotationSequenceAngles=[0 0 0]  RotationSequenceAnglesUnits=deg  RotationMatrix=[1 0 0; 0 1 0; 0 0 1]
  Transform Ornament Front : sm_lib/Frames and Transforms/Rigid Transform  TranslationMethod=Cartesian  TranslationStandardOffset=1  TranslationLengthUnit=m  TranslationStandardAxis=+Z  TranslationCartesianOffset=[max(xy_data_car_side(:,1)) 0 min(xy_data_car_side(:,2))+0.15]  TranslationROffset=0  TranslationROffsetUnits=m  TranslationZOffset=0  TranslationZOffsetUnits=m  TranslationThetaOffset=0  TranslationThetaOffsetUnits=deg  RotationMethod=RotationSequence  RotationAngleUnits=deg  RotationStandardAxis=+Z  RotationAngle=90  RotationArbitraryAxis=[0 0 1]  FollAlignAxisA=+X  BaseAlignAxisA=+Y  FollAlignAxisB=+Y  BaseAlignAxisB=+Z  RotationSequenceAxes=FollowerAxes  RotationSequence=ZXY  RotationSequenceAngles=[90 90 0]  RotationSequenceAnglesUnits=deg  RotationMatrix=[1 0 0; 0 1 0; 0 0 1]
  Transform Ornament Rear : sm_lib/Frames and Transforms/Rigid Transform  TranslationMethod=Cartesian  TranslationStandardOffset=1  TranslationLengthUnit=m  TranslationStandardAxis=+Z  TranslationCartesianOffset=[min(xy_data_car_side(:,1))+0.1 0 min(xy_data_car_side(:,2))+0.15]  TranslationROffset=0  TranslationROffsetUnits=m  TranslationZOffset=0  TranslationZOffsetUnits=m  TranslationThetaOffset=0  TranslationThetaOffsetUnits=deg  RotationMethod=RotationSequence  RotationAngleUnits=deg  RotationStandardAxis=+Z  RotationAngle=90  RotationArbitraryAxis=[0 0 1]  FollAlignAxisA=+X  BaseAlignAxisA=+Y  FollAlignAxisB=+Y  BaseAlignAxisB=+Z  RotationSequenceAxes=FollowerAxes  RotationSequence=ZXY  RotationSequenceAngles=[90 90 180]  RotationSequenceAnglesUnits=deg  RotationMatrix=[1 0 0; 0 1 0; 0 0 1]
  Transform Left Face : sm_lib/Frames and Transforms/Rigid Transform  TranslationMethod=StandardAxis  TranslationStandardOffset=car_track/2-thk_side/2  TranslationLengthUnit=m  TranslationStandardAxis=-Z  TranslationCartesianOffset=[0 0 0]  TranslationROffset=0  TranslationROffsetUnits=m  TranslationZOffset=0  TranslationZOffsetUnits=m  TranslationThetaOffset=0  TranslationThetaOffsetUnits=deg  RotationMethod=None  RotationAngleUnits=deg  RotationStandardAxis=+Z  RotationAngle=0.0  RotationArbitraryAxis=[0 0 1]  FollAlignAxisA=+X  BaseAlignAxisA=+Y  FollAlignAxisB=+Y  BaseAlignAxisB=+Z  RotationSequenceAxes=FollowerAxes  RotationSequence=XYX  RotationSequenceAngles=[0 0 0]  RotationSequenceAnglesUnits=deg  RotationMatrix=[1 0 0; 0 1 0; 0 0 1]
  Transform Right Face : sm_lib/Frames and Transforms/Rigid Transform  TranslationMethod=StandardAxis  TranslationStandardOffset=car_track/2-thk_side/2  TranslationLengthUnit=m  TranslationStandardAxis=+Z  TranslationCartesianOffset=[0 0 0]  TranslationROffset=0  TranslationROffsetUnits=m  TranslationZOffset=0  TranslationZOffsetUnits=m  TranslationThetaOffset=0  TranslationThetaOffsetUnits=deg  RotationMethod=None  RotationAngleUnits=deg  RotationStandardAxis=+Z  RotationAngle=0.0  RotationArbitraryAxis=[0 0 1]  FollAlignAxisA=+X  BaseAlignAxisA=+Y  FollAlignAxisB=+Y  BaseAlignAxisB=+Z  RotationSequenceAxes=FollowerAxes  RotationSequence=XYX  RotationSequenceAngles=[0 0 0]  RotationSequenceAnglesUnits=deg  RotationMatrix=[1 0 0; 0 1 0; 0 0 1]
  FA : PMIOPort  Side=Left
  connections:
  Transform Ornament Front/LConn1 -- Transform Ornament Rear/LConn1 -- FA/RConn1 -- Transform Extrusion Axes/LConn1
  Left Face/RConn1 -- Transform Left Face/RConn1
  Transform Extrusion Axes/RConn1 -- Transform Right Face/LConn1 -- Top Surface/RConn1 -- Transform Left Face/LConn1
  Right Face/RConn1 -- Transform Right Face/RConn1
  Transform Ornament Front/RConn1 -- Ornament Front/RConn1
  Transform Ornament Rear/RConn1 -- Ornament Rear/RConn1

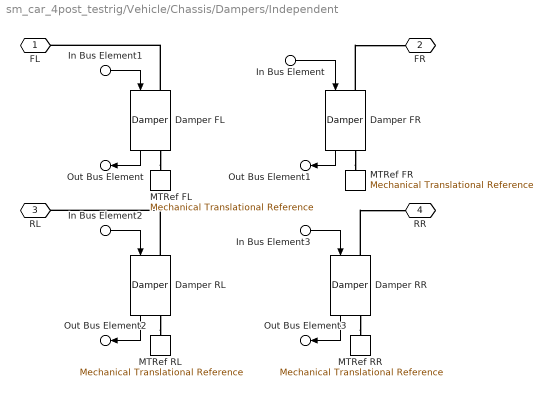
== system sm_car_4post_testrig/Vehicle/Chassis/Dampers/Independent ==
  In Bus Element1 : Inport  PortName=Ctrl  Element=FL
  In Bus Element : Inport  PortName=Ctrl  Element=FR
  In Bus Element2 : Inport  PortName=Ctrl  Element=RL
  In Bus Element3 : Inport  PortName=Ctrl  Element=RR
  Damper FL : sm_car_4post_lib/Damper  Damper=Damper.Front
      settings: SourceProductBaseCode=MS
  Damper FR : sm_car_4post_lib/Damper  Damper=Damper.Front
      settings: SourceProductBaseCode=MS
  Damper RL : sm_car_4post_lib/Damper  Damper=Damper.Rear
      settings: SourceProductBaseCode=MS
  Damper RR : sm_car_4post_lib/Damper  Damper=Damper.Rear
      settings: SourceProductBaseCode=MS
  MTRef FL : fl_lib/Mechanical/Translational Elements/Mechanical Translational Reference
  MTRef FR : fl_lib/Mechanical/Translational Elements/Mechanical Translational Reference
  MTRef RL : fl_lib/Mechanical/Translational Elements/Mechanical Translational Reference
  MTRef RR : fl_lib/Mechanical/Translational Elements/Mechanical Translational Reference
  FL : PMIOPort  Side=Left
  FR : PMIOPort  Port=2  Side=Right
  RL : PMIOPort  Port=3  Side=Left
  RR : PMIOPort  Port=4  Side=Right
  Out Bus Element : Outport  VectorParamsAs1DForOutWhenUnconnected=off  PortName=meas  Element=FL
  Out Bus Element1 : Outport  VectorParamsAs1DForOutWhenUnconnected=off  PortName=meas  Element=FR
  Out Bus Element2 : Outport  VectorParamsAs1DForOutWhenUnconnected=off  PortName=meas  Element=RL
  Out Bus Element3 : Outport  VectorParamsAs1DForOutWhenUnconnected=off  PortName=meas  Element=RR
  wires:
  Damper RR/1 -> Out Bus Element3/1
  Damper RL/1 -> Out Bus Element2/1
  In Bus Element2/1 -> Damper RL/1
  In Bus Element3/1 -> Damper RR/1
  Damper FR/1 -> Out Bus Element1/1
  Damper FL/1 -> Out Bus Element/1
  In Bus Element1/1 -> Damper FL/1
  In Bus Element/1 -> Damper FR/1
  connections:
  Damper FL/RConn1 -- MTRef FL/LConn1
  Damper FL/LConn1 -- FL/RConn1
  Damper RL/RConn1 -- MTRef RL/LConn1
  Damper RL/LConn1 -- RL/RConn1
  Damper RR/RConn1 -- MTRef RR/LConn1
  Damper RR/LConn1 -- RR/RConn1
  Damper FR/RConn1 -- MTRef FR/LConn1
  Damper FR/LConn1 -- FR/RConn1

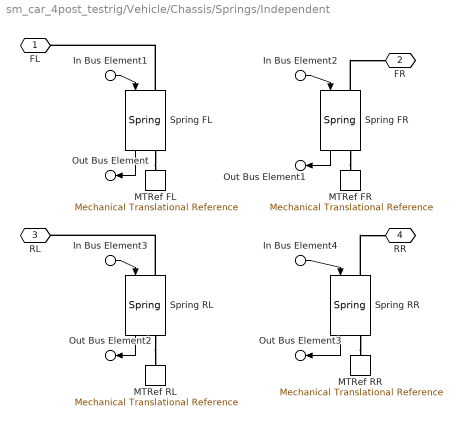
== system sm_car_4post_testrig/Vehicle/Chassis/Springs/Independent ==
  In Bus Element1 : Inport  PortName=Ctrl  Element=FL
  In Bus Element2 : Inport  PortName=Ctrl  Element=FR
  In Bus Element3 : Inport  PortName=Ctrl  Element=RL
  In Bus Element4 : Inport  PortName=Ctrl  Element=RR
  MTRef FL : fl_lib/Mechanical/Translational Elements/Mechanical Translational Reference
  MTRef FR : fl_lib/Mechanical/Translational Elements/Mechanical Translational Reference
  MTRef RL : fl_lib/Mechanical/Translational Elements/Mechanical Translational Reference
  MTRef RR : fl_lib/Mechanical/Translational Elements/Mechanical Translational Reference
  Spring FL : sm_car_4post_lib/Spring  Spring=Spring.Front
      settings: SourceProductBaseCode=MS
  Spring FR : sm_car_4post_lib/Spring  Spring=Spring.Front
      settings: SourceProductBaseCode=MS
  Spring RL : sm_car_4post_lib/Spring  Spring=Spring.Rear
      settings: SourceProductBaseCode=MS
  Spring RR : sm_car_4post_lib/Spring  Spring=Spring.Rear
      settings: SourceProductBaseCode=MS
  FL : PMIOPort  Side=Left
  FR : PMIOPort  Port=2  Side=Right
  RL : PMIOPort  Port=3  Side=Left
  RR : PMIOPort  Port=4  Side=Right
  Out Bus Element : Outport  VectorParamsAs1DForOutWhenUnconnected=off  PortName=meas  Element=FL
  Out Bus Element1 : Outport  VectorParamsAs1DForOutWhenUnconnected=off  PortName=meas  Element=FR
  Out Bus Element2 : Outport  VectorParamsAs1DForOutWhenUnconnected=off  PortName=meas  Element=RL
  Out Bus Element3 : Outport  VectorParamsAs1DForOutWhenUnconnected=off  PortName=meas  Element=RR
  wires:
  Spring RR/1 -> Out Bus Element3/1
  In Bus Element4/1 -> Spring RR/1
  Spring RL/1 -> Out Bus Element2/1
  In Bus Element3/1 -> Spring RL/1
  Spring FR/1 -> Out Bus Element1/1
  In Bus Element2/1 -> Spring FR/1
  Spring FL/1 -> Out Bus Element/1
  In Bus Element1/1 -> Spring FL/1
  connections:
  Spring FL/RConn1 -- MTRef FL/LConn1
  Spring FL/LConn1 -- FL/RConn1
  Spring RL/RConn1 -- MTRef RL/LConn1
  Spring RL/LConn1 -- RL/RConn1
  Spring RR/RConn1 -- MTRef RR/LConn1
  Spring RR/LConn1 -- RR/RConn1
  Spring FR/RConn1 -- MTRef FR/LConn1
  Spring FR/LConn1 -- FR/RConn1

== system sm_car_4post_testrig/Vehicle/Powertrain/Driveline/Gear Reduction Front ==
  note: Note: This configuration requires both shafts to spin at nearly the same speed, which is not realistic for a car. This subsystem should be replaced by a Differential block from Simscape Driveline.
  note: Shaft Flexibility
  Gear Box : fl_lib/Mechanical/Mechanisms/Gear Box  ratio=Driveline.DifferentialF.ratio.Value  t_in_specify=off  t_in_priority=None  t_in=0 N*m  t_in_nominal_specify=off  t_in_nominal_unit=N*m  t_in_nominal_value=1  t_out_specify=off  t_out_priority=None  t_out=0 N*m  t_out_nominal_specify=off  t_out_nominal_unit=N*m  t_out_nominal_value=1
  Rotational Damper : fl_lib/Mechanical/Rotational Elements/Rotational Damper  D=1e3 N*m/(rad/s)  w_specify=off  w_priority=None  w=0 rad/s  w_nominal_specify=off  w_nominal_unit=rad/s  w_nominal_value=1  t_specify=off  t_priority=None  t=0 N*m  t_nominal_specify=off  t_nominal_unit=N*m  t_nominal_value=1
  Rotational Spring : fl_lib/Mechanical/Rotational Elements/Rotational Spring  spr_rate=1e4 N*m/rad  w_specify=off  w_priority=None  w=0 rad/s  w_nominal_specify=off  w_nominal_unit=rad/s  w_nominal_value=1  t_specify=off  t_priority=None  t=0 N*m  t_nominal_specify=off  t_nominal_unit=N*m  t_nominal_value=1  phi_specify=off  phi_priority=High  phi=0 rad  phi_nominal_specify=off  phi_nominal_unit=rad  phi_nominal_value=1
  S1 : PMIOPort  Side=Right
  D : PMIOPort  Port=2  Side=Left
  S2 : PMIOPort  Port=3  Side=Right
  connections:
  Gear Box/LConn1 -- D/RConn1
  Rotational Damper/RConn1 -- S1/RConn1 -- Rotational Spring/RConn1
  Gear Box/RConn1 -- Rotational Damper/LConn1 -- Rotational Spring/LConn1 -- S2/RConn1

== system sm_car_4post_testrig/Vehicle/Powertrain/Driveline/Gear Reduction Rear ==
  note: Shaft Flexibility
  note: Note: This configuration requires both shafts to spin at nearly the same speed, which is not realistic for a car. This subsystem should be replaced by a Differential block from Simscape Driveline.
  Gear Box : fl_lib/Mechanical/Mechanisms/Gear Box  ratio=Driveline.DifferentialR.ratio.Value  t_in_specify=off  t_in_priority=None  t_in=0 N*m  t_in_nominal_specify=off  t_in_nominal_unit=N*m  t_in_nominal_value=1  t_out_specify=off  t_out_priority=None  t_out=0 N*m  t_out_nominal_specify=off  t_out_nominal_unit=N*m  t_out_nominal_value=1
  Rotational Damper : fl_lib/Mechanical/Rotational Elements/Rotational Damper  D=1e3 N*m/(rad/s)  w_specify=off  w_priority=None  w=0 rad/s  w_nominal_specify=off  w_nominal_unit=rad/s  w_nominal_value=1  t_specify=off  t_priority=None  t=0 N*m  t_nominal_specify=off  t_nominal_unit=N*m  t_nominal_value=1
  Rotational Spring : fl_lib/Mechanical/Rotational Elements/Rotational Spring  spr_rate=1e4 N*m/rad  w_specify=off  w_priority=None  w=0 rad/s  w_nominal_specify=off  w_nominal_unit=rad/s  w_nominal_value=1  t_specify=off  t_priority=None  t=0 N*m  t_nominal_specify=off  t_nominal_unit=N*m  t_nominal_value=1  phi_specify=off  phi_priority=High  phi=0 rad  phi_nominal_specify=off  phi_nominal_unit=rad  phi_nominal_value=1
  S1 : PMIOPort  Side=Right
  D : PMIOPort  Port=2  Side=Left
  S2 : PMIOPort  Port=3  Side=Right
  connections:
  Rotational Spring/LConn1 -- Gear Box/RConn1 -- S2/RConn1 -- Rotational Damper/LConn1
  S1/RConn1 -- Rotational Damper/RConn1 -- Rotational Spring/RConn1
  Gear Box/LConn1 -- D/RConn1

== system sm_car_4post_testrig/Vehicle/Powertrain/Driveline/Sensing DriveshaftFL Torque ==
  Ideal Torque Sensor : fl_lib/Mechanical/Mechanical Sensors/Ideal Torque Sensor
  PS-Simulink Converter : nesl_utility/PS-Simulink Converter  PhysicalDomain=network_engine_domain  SubClassName=ps_output  LeftPortType=input  RightPortType=output  PseudoPeriodic=off  Frequencies=[]  Unit=N*m  AffineConversion=off
      settings: SourceProductBaseCode=PW,SS
  C : PMIOPort  Side=Right
  R : PMIOPort  Port=2  Side=Left
  M : Outport  VectorParamsAs1DForOutWhenUnconnected=off
  wires:
  PS-Simulink Converter/1 -> M/1
  connections:
  Ideal Torque Sensor/RConn2 -- PS-Simulink Converter/LConn1
  R/RConn1 -- Ideal Torque Sensor/LConn1
  Ideal Torque Sensor/RConn1 -- C/RConn1

== system sm_car_4post_testrig/Vehicle/Powertrain/Driveline/Sensing DriveshaftFR Torque ==
  Ideal Torque Sensor : fl_lib/Mechanical/Mechanical Sensors/Ideal Torque Sensor
  PS-Simulink Converter : nesl_utility/PS-Simulink Converter  PhysicalDomain=network_engine_domain  SubClassName=ps_output  LeftPortType=input  RightPortType=output  PseudoPeriodic=off  Frequencies=[]  Unit=N*m  AffineConversion=off
      settings: SourceProductBaseCode=PW,SS
  C : PMIOPort  Side=Right
  R : PMIOPort  Port=2  Side=Left
  M : Outport  VectorParamsAs1DForOutWhenUnconnected=off
  wires:
  PS-Simulink Converter/1 -> M/1
  connections:
  Ideal Torque Sensor/RConn1 -- C/RConn1
  R/RConn1 -- Ideal Torque Sensor/LConn1
  Ideal Torque Sensor/RConn2 -- PS-Simulink Converter/LConn1

== system sm_car_4post_testrig/Vehicle/Powertrain/Driveline/Sensing DriveshaftRL Torque ==
  Ideal Torque Sensor : fl_lib/Mechanical/Mechanical Sensors/Ideal Torque Sensor
  PS-Simulink Converter : nesl_utility/PS-Simulink Converter  PhysicalDomain=network_engine_domain  SubClassName=ps_output  LeftPortType=input  RightPortType=output  PseudoPeriodic=off  Frequencies=[]  Unit=N*m  AffineConversion=off
      settings: SourceProductBaseCode=PW,SS
  C : PMIOPort  Side=Right
  R : PMIOPort  Port=2  Side=Left
  M : Outport  VectorParamsAs1DForOutWhenUnconnected=off
  wires:
  PS-Simulink Converter/1 -> M/1
  connections:
  Ideal Torque Sensor/RConn1 -- C/RConn1
  R/RConn1 -- Ideal Torque Sensor/LConn1
  Ideal Torque Sensor/RConn2 -- PS-Simulink Converter/LConn1

== system sm_car_4post_testrig/Vehicle/Powertrain/Driveline/Sensing DriveshaftRR Torque ==
  Ideal Torque Sensor : fl_lib/Mechanical/Mechanical Sensors/Ideal Torque Sensor
  PS-Simulink Converter : nesl_utility/PS-Simulink Converter  PhysicalDomain=network_engine_domain  SubClassName=ps_output  LeftPortType=input  RightPortType=output  PseudoPeriodic=off  Frequencies=[]  Unit=N*m  AffineConversion=off
      settings: SourceProductBaseCode=PW,SS
  C : PMIOPort  Side=Right
  R : PMIOPort  Port=2  Side=Left
  M : Outport  VectorParamsAs1DForOutWhenUnconnected=off
  wires:
  PS-Simulink Converter/1 -> M/1
  connections:
  Ideal Torque Sensor/RConn2 -- PS-Simulink Converter/LConn1
  R/RConn1 -- Ideal Torque Sensor/LConn1
  Ideal Torque Sensor/RConn1 -- C/RConn1
